simulink model "MRAS_IR2_Ld_Lq_U_comp_dt2_new"  (R2018a)
settings: Solver=ode23t  StartTime=0.0  StopTime=0.3  MaxStep=1e-5  RelTol=1e-4  EnableMultiTasking=on
libraries: powerlib x10, powerlib_meascontrol x10, simulink x1
settings Model: Creator=Алексей  LastModifiedBy=Len_comp
settings SolverCC: ZeroCrossControl=DisableAll  ZeroCrossAlgorithm=Adaptive
settings DataIOCC: SaveFormat=Array  SaveOutput=off  DSMLogging=off  SaveTime=off
settings OptimizationCC: LifeSpan=inf
settings DebuggingCC: UnderspecifiedInitializationDetection=Classic  MergeDetectMultiDrivingBlocksExec=none  SolverPrmCheckMsg=warning  AllowSymbolicDim=off  SFUnexpectedBacktrackingDiag=warning  SFNoUnconditionalDefaultTransitionDiag=warning  SFExecutionAtInitializationDiag=none
settings HardwareCC: ProdBitPerPointer=32  ProdBitPerSizeT=32  ProdBitPerPtrDiffT=32  ProdLargestAtomicFloat=None  ProdIntDivRoundTo=Undefined  ProdEndianess=Unspecified  ProdWordSize=32  ProdHWDeviceType=32-bit Generic
settings ModelReferenceCC: PropagateSignalLabelsOutOfModel=off
settings CodeAppCC: StateflowObjectComments=on
settings GRTTargetCC: TargetLangStandard=C89/C90 (ANSI)  GeneratePreprocessorConditionals=Disable all
settings ConfigComp: CovMetricSettings=dw  CovHtmlReporting=on  CovSaveCumulativeToWorkspaceVar=on  CovSaveSingleToWorkspaceVar=on  CovExternalEMLEnable=off  CovSFcnEnable=off
settings SimscapeCC: SimscapeNormalizeSystem=off

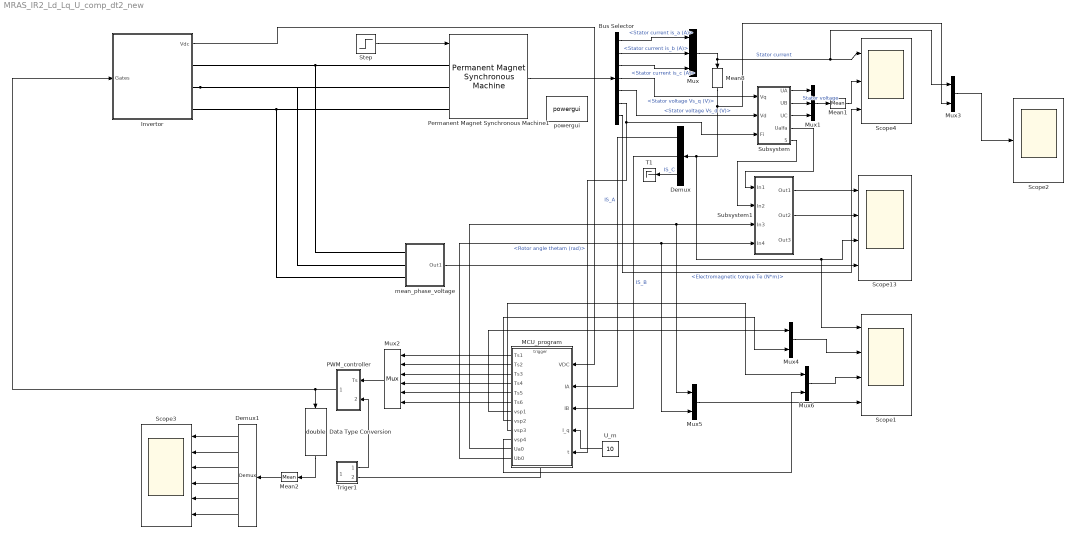
== system MRAS_IR2_Ld_Lq_U_comp_dt2_new ==
  Bus Selector : BusSelector  OutputSignals=Stator current is_a (A),Stator current is_b (A),Stator current is_c (A),Stator voltage Vs_q (V),Stator voltage Vs_d (V),Rotor angle thetam (rad),Electromagnetic torque Te (N*m)
  Data Type Conversion : DataTypeConversion  OutDataTypeStr=double
  Demux : Demux  Outputs=3
  Demux1 : Demux  Outputs=6
  Invertor : Subsystem
  MCU_program : MATLAB Function  TreatAsAtomicUnit=on
  Mean1 : powerlib_meascontrol/Measurements/Mean  Freq=10000  Vinit=0  Ts=0
  Mean2 : powerlib_meascontrol/Measurements/Mean  Freq=10000  Vinit=0  Ts=0
  Mean8 : powerlib_meascontrol/Measurements/Mean  Freq=20000  Vinit=0  Ts=0
  Mux : Mux  Inputs=3
  Mux1 : Mux  Inputs=3
  Mux2 : Mux  Inputs=6
  Mux{3..6} (4 alike) : Mux  Inputs=2
  PWM_controller : Subsystem
  Permanent Magnet Synchronous Machine1 : powerlib/Machines/Permanent Magnet Synchronous Machine  NbPhases=3  FluxDistribution=Sinusoidal  RotorType=Round  MechanicalLoad=Speed w  PresetModel=No  ShowDetailedParameters=on  MeasurementBus=off  Resistance=0.04  Inductance=8.5e-3  dqInductances=[44e-3,39.8e-3]  La=15e-6  MachineConstant=Flux linkage established by magnets (V.s)  Flux=0.0345  VoltageCst=6.2576  TorqueCst=0.05175  Flat=120  Mechanical=[2e4 3e-03 1 0]  PolePairs=1  InitialConditions=[0,0, 0,0]  InitialConditions5ph=[0 0 0 0 0 0]  TsPowergui=0  TsBlock=-1  RefAngle=Aligned with phase A axis (original Park)
      settings: SourceProductName=Simscape Power Systems
  Scope1 : Scope  NumInputPorts=4
  Scope13 : Scope  NumInputPorts=4
  Scope2 : Scope
  Scope3 : Scope  NumInputPorts=6
  Scope4 : Scope  NumInputPorts=3
  Step : Step  Time=0.025  Before=500  After=50  SampleTime=0
  Subsystem : Subsystem
  Subsystem1 : Subsystem
  T1 : Terminator
  Triger1 : Subsystem
  U_m : Constant  Value=10
  mean_phase_voltage : Subsystem
  powergui : powerlib/powergui  Priority=1  SimulationMode=Continuous  SampleTime=50e-6  frequency=60  Iterations=50  frequencyindice=0  Pbase=100e6  ErrMax=1e-4  UnitsV=kV  UnitsW=MW  buscounter=0  FunctionMessages=off  echomessages=off  EnableUseOfTLC=off  CurrentSourceSwitches=on  DisableSnubberDevices=off  DisableRonSwitches=off  DisableVfSwitches=off  DisplayEquations=off  SolverType=Tustin  Interpol=off  ExternalGateDelay=off  methode=off  Ts=0  x0status=blocks  SPID=off  SwTol=0  HookPort=off  RestoreLinks=warning  ResistiveCurrentMeasurement=off  Frange=[0:2:500]  Ylog=off  Xlog=on  ShowGrid=off  save=off  variable=ZData  structure=SD2  ZoomFFT=on  StartTime=0.7  cycles=10  DisplayStyle=4  fundamental=382  FreqAxis=off  MaxFrequency=50000  frequencyindicesteady=1  RmsSteady=1  display=off
  wires:
  Demux/1 -> MCU_program/2(IA)  "IS_A"
  Demux/2 -> MCU_program/3(IB)  "IS_B"
  Permanent Magnet Synchronous Machine1/1 -> Bus Selector/1
  Bus Selector/1 -> Mux/1  "<Stator current is_a (A)>"
  Bus Selector/2 -> Mux/2  "<Stator current is_b (A)>"
  Bus Selector/3 -> Mux/3  "<Stator current is_c (A)>"
  Bus Selector/4 -> Subsystem/1(Vq)  "<Stator voltage Vs_q (V)>"
  Bus Selector/5 -> Subsystem/2(Vd)  "<Stator voltage Vs_d (V)>"
  Subsystem/2(UB) -> Mux1/2
  Subsystem/3(UC) -> Mux1/3
  Subsystem/1(UA) -> Mux1/1
  Mux/1 -> Mean8/1, Mux3/1, Scope4/1  "Stator current"
  Mux1/1 -> Mean1/1  "Stator voltage"
  Step/1 -> Permanent Magnet Synchronous Machine1/1
  MCU_program/1(Ts1) -> Mux2/1
  MCU_program/2(Ts2) -> Mux2/2
  MCU_program/3(Ts3) -> Mux2/3
  MCU_program/4(Ts4) -> Mux2/4
  MCU_program/5(Ts5) -> Mux2/5
  MCU_program/6(Ts6) -> Mux2/6
  Mux2/1 -> PWM_controller/1(Ts)
  Triger1/1(1) -> PWM_controller/2(pila)
  PWM_controller/1(Tss) -> Invertor/1(Gates), Data Type Conversion/1
  Triger1/2(2) -> MCU_program/Trigger
  Invertor/1(Vdc) -> MCU_program/1(VDC)
  Demux/3 -> T1/1  "IS_C"
  U_m/1 -> MCU_program/4(I_q)
  Mean8/1 -> Mux3/2, Scope1/1, Scope13/3, Demux/1
  Demux1/1 -> Scope3/1
  Demux1/3 -> Scope3/3
  Demux1/2 -> Scope3/2
  Demux1/4 -> Scope3/4
  Demux1/5 -> Scope3/5
  Demux1/6 -> Scope3/6
  mean_phase_voltage/1(Out1) -> Scope13/4
  Subsystem/4(Ualfa) -> Subsystem1/1(In1)
  Subsystem/5(Ubeta) -> Subsystem1/2(In2)
  MCU_program/11(Ua0) -> Mux5/1, Subsystem1/3(In3)
  MCU_program/12(Ub0) -> Subsystem1/4(In4), Mux5/2
  Subsystem1/1(Out1) -> Scope13/1
  Subsystem1/2(Out2) -> Scope13/2
  MCU_program/7(vsp1) -> Mux4/1
  MCU_program/8(vsp2) -> Mux4/2
  MCU_program/9(vsp3) -> Mux6/1
  Mux3/1 -> Scope2/1
  Mean1/1 -> Scope4/2
  Mean2/1 -> Demux1/1
  Data Type Conversion/1 -> Mean2/1
  MCU_program/10(vsp4) -> Mux6/2
  Mux5/1 -> Scope1/4
  Mux6/1 -> Scope1/3
  Mux4/1 -> Scope1/2
  Bus Selector/6 -> Subsystem/3(Fi), MCU_program/5(t)  "<Rotor angle thetam (rad)>"
  Bus Selector/7 -> Scope4/3  "<Electromagnetic torque Te (N*m)>"
  connections:
  Permanent Magnet Synchronous Machine1/LConn1 -- mean_phase_voltage/LConn1 -- Invertor/RConn1
  Invertor/RConn2 -- mean_phase_voltage/LConn2 -- Permanent Magnet Synchronous Machine1/LConn2
  Invertor/RConn3 -- mean_phase_voltage/LConn3 -- Permanent Magnet Synchronous Machine1/LConn3

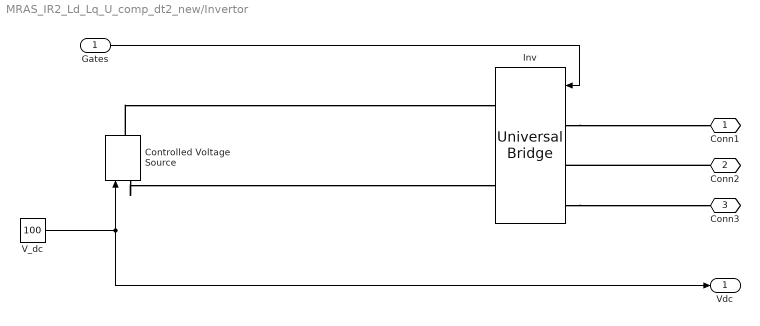
== system MRAS_IR2_Ld_Lq_U_comp_dt2_new/Invertor ==
  Gates : Inport
  Controlled Voltage Source : powerlib/Electrical Sources/Controlled Voltage Source  Initialize=on  Source_Type=AC  Amplitude=0  Phase=0  Frequency=0  Measurements=None
  Inv : powerlib/Power Electronics/Universal Bridge  Arms=3  SnubberResistance=1e9  SnubberCapacitance=inf  Device=IGBT / Diodes  Ron=1e-6  Lon=0  ForwardVoltages="[  0 0  ]"  ForwardVoltage=0  GTOparameters=[ 10e-6 , 20e-6 ]  IGBTparameters=[ 1e-7 , 1e-7 ]  Measurements=None  Measurements_2=None  converterType=Rectifier
  "V_dc " : Constant  Value=100
  Conn1 : PMIOPort  Side=Right
  Conn2 : PMIOPort  Port=2  Side=Right
  Conn3 : PMIOPort  Port=3  Side=Right
  Vdc : Outport
  wires:
  Gates/1 -> Inv/1
  "V_dc "/1 -> Controlled Voltage Source/1, Vdc/1
  connections:
  Controlled Voltage Source/RConn1 -- Inv/RConn1
  Conn2/RConn1 -- Inv/LConn2
  Controlled Voltage Source/LConn1 -- Inv/RConn2
  Inv/LConn3 -- Conn3/RConn1
  Inv/LConn1 -- Conn1/RConn1

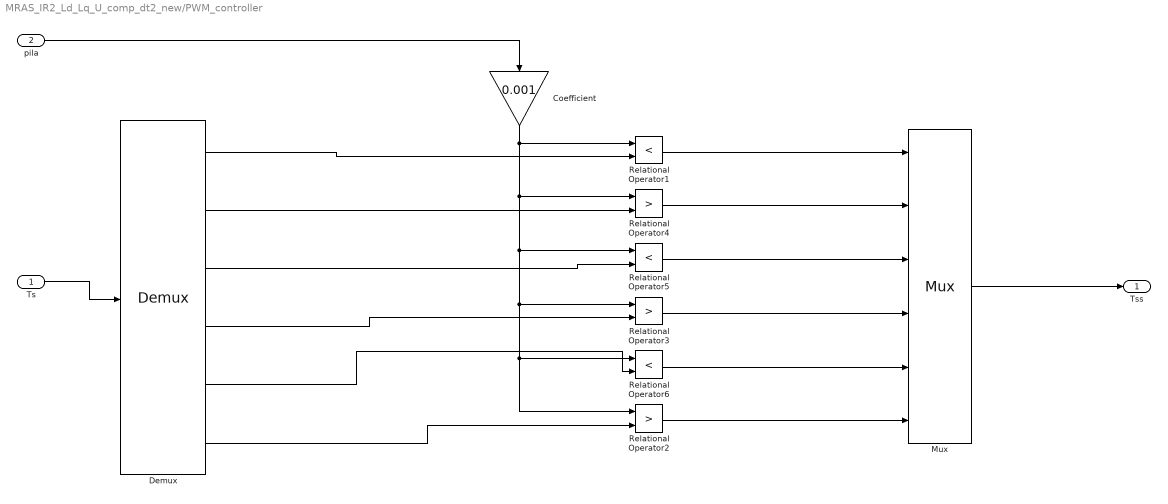
== system MRAS_IR2_Ld_Lq_U_comp_dt2_new/PWM_controller ==
  Ts : Inport
  pila : Inport  Port=2
  Coefficient : Gain  Gain=0.001
  Demux : Demux  Outputs=6
  Mux : Mux  Inputs=6
  Relational Operator1 : RelationalOperator  Operator=<  OutDataTypeStr=boolean  RndMeth=Nearest
  Relational Operator2 : RelationalOperator  Operator=>  OutDataTypeStr=boolean  RndMeth=Nearest
  Relational Operator3 : RelationalOperator  Operator=>  OutDataTypeStr=boolean  RndMeth=Nearest
  Relational Operator4 : RelationalOperator  Operator=>  OutDataTypeStr=boolean  RndMeth=Nearest
  Relational Operator5 : RelationalOperator  Operator=<  OutDataTypeStr=boolean  RndMeth=Nearest
  Relational Operator6 : RelationalOperator  Operator=<  OutDataTypeStr=boolean  RndMeth=Nearest
  Tss : Outport
  wires:
  Relational Operator4/1 -> Mux/2
  Demux/4 -> Relational Operator3/2
  Demux/6 -> Relational Operator2/2
  Relational Operator3/1 -> Mux/4
  Relational Operator2/1 -> Mux/6
  Ts/1 -> Demux/1
  Coefficient/1 -> Relational Operator3/1, Relational Operator2/1, Relational Operator6/1, Relational Operator5/1, Relational Operator4/1, Relational Operator1/1
  Relational Operator1/1 -> Mux/1
  Relational Operator5/1 -> Mux/3
  Relational Operator6/1 -> Mux/5
  Demux/1 -> Relational Operator1/2
  Demux/3 -> Relational Operator5/2
  Demux/5 -> Relational Operator6/2
  Demux/2 -> Relational Operator4/2
  pila/1 -> Coefficient/1
  Mux/1 -> Tss/1

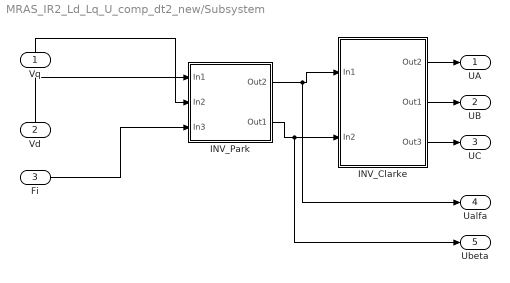
== system MRAS_IR2_Ld_Lq_U_comp_dt2_new/Subsystem ==
  Vq : Inport
  Vd : Inport  Port=2
  Fi : Inport  Port=3
  INV_Clarke : Subsystem
  INV_Park : Subsystem
  UA : Outport
  UB : Outport  Port=2
  UC : Outport  Port=3
  Ualfa : Outport  Port=4
  Ubeta : Outport  Port=5
  wires:
  INV_Clarke/2(Out1) -> UB/1
  INV_Park/1(Out2) -> Ualfa/1, INV_Clarke/1(In1)
  INV_Clarke/1(Out2) -> UA/1
  INV_Park/2(Out1) -> Ubeta/1, INV_Clarke/2(In2)
  INV_Clarke/3(Out3) -> UC/1
  Fi/1 -> INV_Park/3(In3)
  Vd/1 -> INV_Park/1(In1)
  Vq/1 -> INV_Park/2(In2)

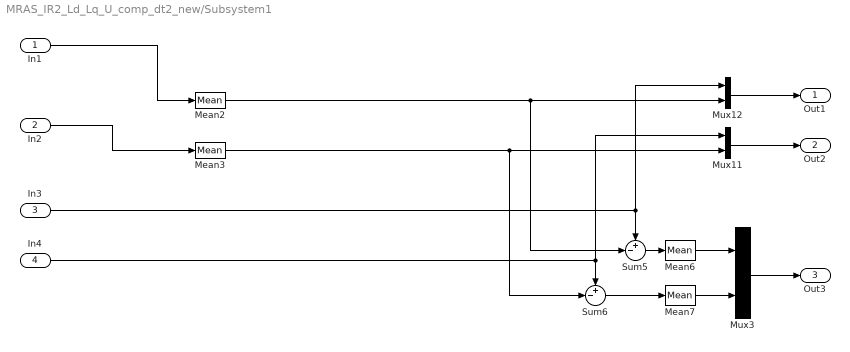
== system MRAS_IR2_Ld_Lq_U_comp_dt2_new/Subsystem1 ==
  In1 : Inport
  In2 : Inport  Port=2
  In3 : Inport  Port=3
  In4 : Inport  Port=4
  Mean2 : powerlib_meascontrol/Measurements/Mean  Freq=10000  Vinit=0  Ts=0
  Mean3 : powerlib_meascontrol/Measurements/Mean  Freq=10000  Vinit=0  Ts=0
  Mean6 : powerlib_meascontrol/Measurements/Mean  Freq=20000  Vinit=0  Ts=0
  Mean7 : powerlib_meascontrol/Measurements/Mean  Freq=20000  Vinit=0  Ts=0
  Mux11 : Mux  Inputs=2
  Mux12 : Mux  Inputs=2
  Mux3 : Mux  Inputs=2
  Sum5 : Sum  Inputs=+-|
  Sum6 : Sum  Inputs=+-|
  Out1 : Outport
  Out2 : Outport  Port=2
  Out3 : Outport  Port=3
  wires:
  In4/1 -> Mux11/1, Sum6/1
  Mean7/1 -> Mux3/2
  Sum6/1 -> Mean7/1
  Mean2/1 -> Sum5/2, Mux12/2
  Mean3/1 -> Sum6/2, Mux11/2
  Mean6/1 -> Mux3/1
  Mux11/1 -> Out2/1
  Sum5/1 -> Mean6/1
  In3/1 -> Sum5/1, Mux12/1
  In1/1 -> Mean2/1
  In2/1 -> Mean3/1
  Mux12/1 -> Out1/1
  Mux3/1 -> Out3/1

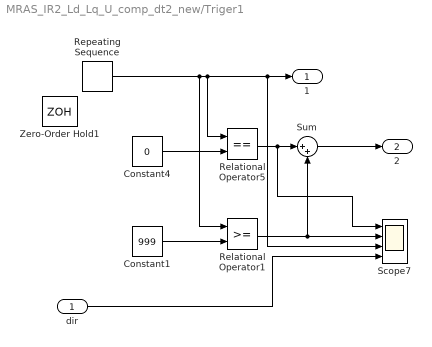
== system MRAS_IR2_Ld_Lq_U_comp_dt2_new/Triger1 ==
  dir : Inport
  Constant1 : Constant  Value=999
  Constant4 : Constant  Value=0
  Relational Operator1 : RelationalOperator  OutDataTypeStr=boolean  RndMeth=Nearest
  Relational Operator5 : RelationalOperator  Operator===  OutDataTypeStr=boolean  RndMeth=Nearest
  Repeating Sequence : simulink/Sources/Repeating Sequence  rep_seq_t=[0 2.5e-5 5e-5]  rep_seq_y=[0 1000 0]
  Scope7 : Scope  NumInputPorts=4
  Sum : Sum  Inputs=|++
  Zero-Order Hold1 : ZeroOrderHold  SampleTime=5e-9
  1 : Outport
  2 : Outport  Port=2
  wires:
  Repeating Sequence/1 -> Relational Operator1/1, Relational Operator5/1, Scope7/3, 1/1
  Constant4/1 -> Relational Operator5/2
  Sum/1 -> 2/1
  Constant1/1 -> Relational Operator1/2
  Relational Operator5/1 -> Scope7/1, Sum/1
  Relational Operator1/1 -> Scope7/2, Sum/2
  dir/1 -> Scope7/4

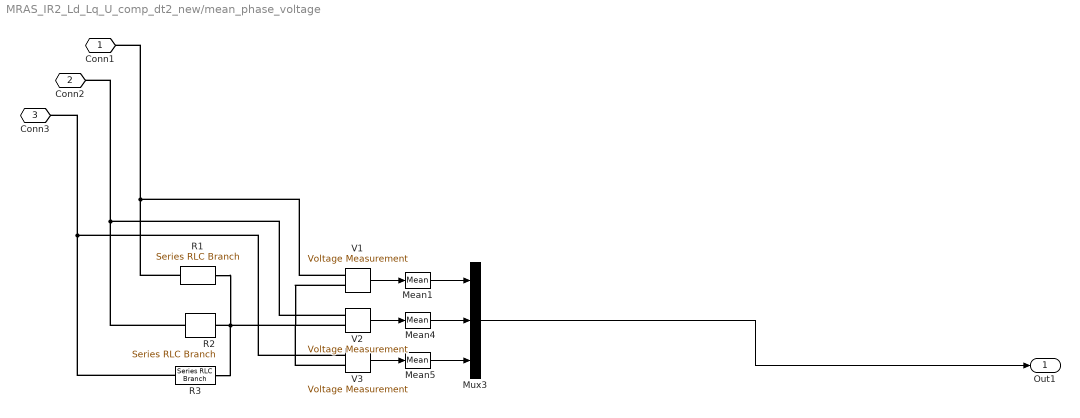
== system MRAS_IR2_Ld_Lq_U_comp_dt2_new/mean_phase_voltage ==
  Mean1 : powerlib_meascontrol/Measurements/Mean  Freq=10000  Vinit=0  Ts=0
  Mean4 : powerlib_meascontrol/Measurements/Mean  Freq=10000  Vinit=0  Ts=0
  Mean5 : powerlib_meascontrol/Measurements/Mean  Freq=10000  Vinit=0  Ts=0
  Mux3 : Mux  Inputs=3
  R1 : powerlib/Elements/Series RLC Branch  LConnTagsString=__new0  RConnTagsString=__new0  BranchType=R  Resistance=1e6  Inductance=1e-3  SetiL0=off  InitialCurrent=0  Capacitance=1e-6  Setx0=off  InitialVoltage=0  Measurements=None
  R2 : powerlib/Elements/Series RLC Branch  LConnTagsString=__new0  RConnTagsString=__new0  BranchType=R  Resistance=1e6  Inductance=1e-3  SetiL0=off  InitialCurrent=0  Capacitance=1e-6  Setx0=off  InitialVoltage=0  Measurements=None
  R3 : powerlib/Elements/Series RLC Branch  LConnTagsString=__new0  RConnTagsString=__new0  BranchType=R  Resistance=1e6  Inductance=1e-3  SetiL0=off  InitialCurrent=0  Capacitance=1e-6  Setx0=off  InitialVoltage=0  Measurements=None
  V1 : powerlib/Measurements/Voltage Measurement  PhasorSimulation=off  OutputType=Complex  PSBequivalent=0
  V2 : powerlib/Measurements/Voltage Measurement  PhasorSimulation=off  OutputType=Complex  PSBequivalent=0
  V3 : powerlib/Measurements/Voltage Measurement  PhasorSimulation=off  OutputType=Complex  PSBequivalent=0
  Conn1 : PMIOPort  Side=Left
  Conn2 : PMIOPort  Port=2  Side=Left
  Conn3 : PMIOPort  Port=3  Side=Left
  Out1 : Outport
  wires:
  V2/1 -> Mean4/1
  Mean1/1 -> Mux3/1
  V3/1 -> Mean5/1
  Mean4/1 -> Mux3/2
  Mean5/1 -> Mux3/3
  V1/1 -> Mean1/1
  Mux3/1 -> Out1/1
  connections:
  R3/LConn1 -- Conn3/RConn1 -- V3/LConn1
  R2/LConn1 -- Conn2/RConn1 -- V2/LConn1
  R3/RConn1 -- V3/LConn2 -- V1/LConn2 -- V2/LConn2 -- R1/RConn1 -- R2/RConn1
  R1/LConn1 -- Conn1/RConn1 -- V1/LConn1

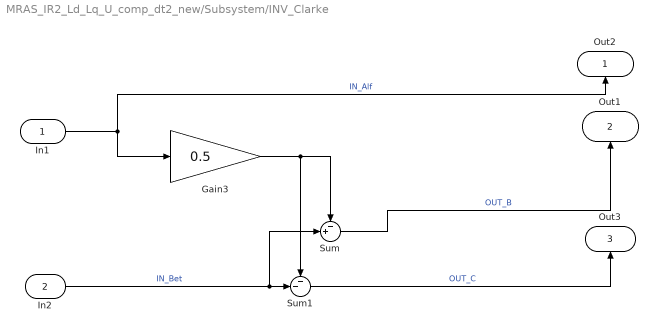
== system MRAS_IR2_Ld_Lq_U_comp_dt2_new/Subsystem/INV_Clarke ==
  In1 : Inport
  In2 : Inport  Port=2
  Gain3 : Gain  Gain=0.5
  Sum : Sum  Inputs=-+|
  Sum1 : Sum  Inputs=--|
  Out2 : Outport
  Out1 : Outport  Port=2
  Out3 : Outport  Port=3
  wires:
  Sum/1 -> Out1/1  "OUT_B"
  In2/1 -> Sum/2, Sum1/2  "IN_Bet"
  In1/1 -> Out2/1, Gain3/1  "IN_Alf"
  Sum1/1 -> Out3/1  "OUT_C"
  Gain3/1 -> Sum1/1, Sum/1

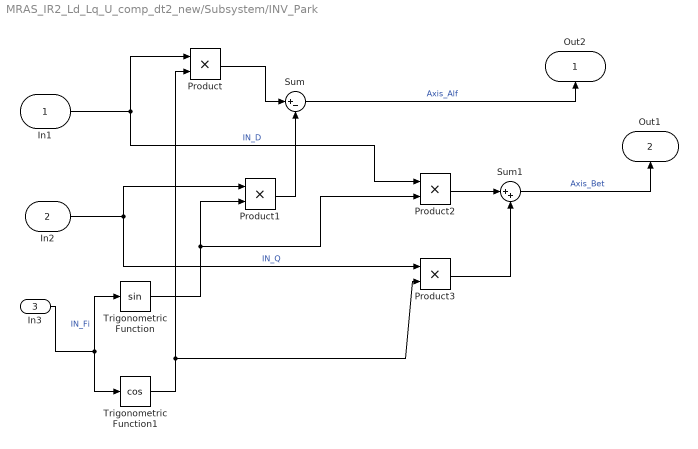
== system MRAS_IR2_Ld_Lq_U_comp_dt2_new/Subsystem/INV_Park ==
  In1 : Inport
  In2 : Inport  Port=2
  In3 : Inport  Port=3
  Product{,1..3} (4 alike) : Product
  Sum : Sum  Inputs=|+-
  Sum1 : Sum  Inputs=|++
  Trigonometric Function : Trigonometry
  Trigonometric Function1 : Trigonometry  Operator=cos
  Out2 : Outport
  Out1 : Outport  Port=2
  wires:
  Sum1/1 -> Out1/1  "Axis_Bet"
  In2/1 -> Product1/1, Product3/1  "IN_Q"
  In1/1 -> Product2/1, Product/1  "IN_D"
  Sum/1 -> Out2/1  "Axis_Alf"
  In3/1 -> Trigonometric Function1/1, Trigonometric Function/1  "IN_Fi"
  Trigonometric Function1/1 -> Product/2, Product3/2
  Trigonometric Function/1 -> Product2/2, Product1/2
  Product1/1 -> Sum/2
  Product/1 -> Sum/1
  Product2/1 -> Sum1/1
  Product3/1 -> Sum1/2

== matlab function MRAS_IR2_Ld_Lq_U_comp_dt2_new/MCU_program ==
  data: VDC input; IA input; IB input; Ts1 output; Ts2 output; Ts3 output; Ts4 output; Ts5 output; Ts6 output; I_q input; vsp1 output; vsp2 output; vsp3 output; vsp4 output; Ua0 output; Ub0 output; t input
  events: trigger input RISING_EDGE_EVENT
function [Ts1,Ts2,Ts3,Ts4,Ts5,Ts6,vsp1,vsp2,vsp3,vsp4,Ua0,Ub0] = fcn(VDC,IA,IB,I_q,t)
%время 1/2 ШИМ периода
dt=25e-6;

dead=0.00;
dtc =0.00;
dtc=dtc/(dt*1e6);

Uvt=0;
Uvd=0;
w=50;

kuqp =0.5;
kudp =0.5;
kuqi =1333;
kudi =1333;

%persistent tet;
persistent dir;
persistent IAp;
persistent IBp;
persistent ICp;

persistent Udint;
persistent Uqint;

%заполнение начальных значений static переменным (persistent здесь)

%if isempty(tet)
%    tet=pi/2;
%end; 

if isempty(dir)
    dir=1;
end; 
if isempty(IAp)
    IAp=0;
end; 
if isempty(IBp)
    IBp=0;
end; 
if isempty(ICp)
    ICp=0;
end; 
if isempty(Udint)
    Udint=0;
end; 
if isempty(Uqint)
    Uqint=0;
end; 




%tet=tet+w*dt;
tet = t;
while (tet > 2*pi)
    tet = tet-2*pi;
end;

Ialfa=IA;
Ibeta=(2*IB+IA)/1.7320508;
Id=Ialfa*cos(tet)+Ibeta*sin(tet);
Iq=Ibeta*cos(tet)-Ialfa*sin(tet); 


%ПИ-регулятор для напряжения по оси Ку
diq=I_q-Iq;
Uqpr=diq*kuqp;
Uqint=Uqint+diq*kuqi*dt;
U_q = Uqpr+Uqint;
%ПИ-регулятор для напряжения по оси Дэ
did=0-Id;
Udpr=did*kudp;
Udint=Udint+did*kudi*dt;
U_d = Udpr+Udint;


%U_d = 0;
%U_q = 2;



Ua0=U_d*cos(tet)-U_q*sin(tet);
Ub0=U_d*sin(tet)+U_q*cos(tet);



%Ua0k=Ua0+(SIA-0.5*SIB-0.5*SIC)*(dead/(2*dt*1e6))*VDC*2/3;
%Ub0k=Ub0+(SIB-SIC)*(dead/(2*dt*1e6))*(sqrt(3)/2)*VDC*2/3;
Ua0k=Ua0;
Ub0k=Ub0;

%{
vref1=sqrt(Ua0^2+Ub0^2);

Ua0k=Ua0k+(sign(IA)-0.5*sign(IB)-0.5*sign(-IA-IB))*0.5*Uvd*(2/3-vref1/VDC);
Ub0k=Ub0k+(sign(IB)-sign(-IA-IB))*0.5*Uvd*(2/3-vref1/VDC)*(sqrt(3)/2);

Ua0k=Ua0k+(sign(IA)-0.5*sign(IB)-0.5*sign(-IA-IB))*Uvt*(1/3+0.41*vref1/VDC);
Ub0k=Ub0k+(sign(IB)-sign(-IA-IB))*Uvt*(1/3+0.41*vref1/VDC)*(sqrt(3)/2);
%}


vrefa=sqrt(Ua0k^2+Ub0k^2);

vphase=acos(Ua0k/vrefa)*sign(Ub0k)+(sign(Ub0k)-1)*(-pi);

if(vrefa>(2/3)*VDC)
  vrefa=(2/3)*VDC;
end
%вывод на осциллографы



vsp1=tet;
vsp2=vphase;
vsp3=U_d;
vsp4=U_q;

%алгоритм формирования векторной ШИМ  мертвым веменем dead [мкс]
dead=dead/(dt*1e6);
a=vphase;
v2=vrefa*1.5;

%v2=v2+2;
if a>=0 && a<pi/3 
    n=1;
elseif  a>=pi/3 && a<2*pi/3 
    n=2;
elseif  a>=2*pi/3 && a<pi 
    n=3;
elseif  a>=pi && a<4*pi/3 
    n=4;
elseif  a>=4*pi/3 && a<5*pi/3 
    n=5;
else n=6;

end

a_cor=a-(n-1)*pi/3;

T1 = (v2/VDC)*sin(pi/3-a_cor)/sin(pi/3);
T2 = (v2/VDC)*sin(a_cor)/sin(pi/3);
T0=1-T1-T2;
Ta1=0; Ta3=0; Ta5=0; 
switch n
    case 1
        
        Ta1=T1+T2+T0/2;
        
        Ta3=T2+T0/2;
       
        Ta5=T0/2;
       
    case 2
        
        Ta1=T1+T0/2;
        
        Ta3=T1+T2+T0/2;
    
        Ta5=T0/2;       
        
    case 3
        
        Ta1=T0/2;
       
        Ta3=T1+T2+T0/2;
       
        Ta5=T2+T0/2;    
        
    case 4
        
        Ta1=T0/2;
       
        Ta3=T1+T0/2;
       
        Ta5=T1+T2+T0/2;   
       
    case 5
        
        Ta1=T2+T0/2;
        
        Ta3=T0/2;
        
        Ta5=T1+T2+T0/2;     
        
    case 6
        
        Ta1=T1+T2+T0/2;
        
        Ta3=T0/2;
     
        Ta5=T1+T0/2;    
        
end;

if(IA>-0.0)
    Ta1=(Ta1*VDC+Uvd)/(VDC-Uvt+Uvd);
elseif(IA<=0.0)
    Ta1=(Ta1*VDC-Uvt)/(VDC-Uvt+Uvd);
end;

if(IB>-0.0)
    Ta3=(Ta3*VDC+Uvd)/(VDC-Uvt+Uvd);
elseif(IB<0.0)
    Ta3=(Ta3*VDC-Uvt)/(VDC-Uvt+Uvd);
end;

if((-IA-IB)>-0.0)
    Ta5=(Ta5*VDC+Uvd)/(VDC-Uvt+Uvd);
elseif((-IA-IB)<0.0)
    Ta5=(Ta5*VDC-Uvt)/(VDC-Uvt+Uvd);
end;


Ts1=(Ta1)+dead/2; 
Ts3=(Ta3)+dead/2; 
Ts5=(Ta5)+dead/2;
Ts2=(Ta1)-dead/2; 
Ts4=(Ta3)-dead/2; 
Ts6=(Ta5)-dead/2;

%{
if(dir==1)
    Ts1=(Ta1); 
    Ts3=(Ta3); 
    Ts5=(Ta5);
    Ts2=(Ta1)+dead; 
    Ts4=(Ta3)+dead; 
    Ts6=(Ta5)+dead;
else
    Ts1=(Ta1)-dead; 
    Ts3=(Ta3)-dead; 
    Ts5=(Ta5)-dead;
    Ts2=(Ta1); 
    Ts4=(Ta3); 
    Ts6=(Ta5);    
end;
%}

if (IA>-0.0)
    Ts1=Ts1+dtc/2;
    Ts2=Ts2+dtc/2;
elseif (IA<0.0)
    Ts1=Ts1-dtc/2;
    Ts2=Ts2-dtc/2;           
end;
if (IB>-0.0)
    Ts3=Ts3+dtc/2;
    Ts4=Ts4+dtc/2;
elseif(IB<0.0)
    Ts3=Ts3-dtc/2;
    Ts4=Ts4-dtc/2; 
end;  
if ((-IA-IB)>-0.0)
    Ts5=Ts5+dtc/2;
    Ts6=Ts6+dtc/2;
elseif((-IA-IB)<0.0)
    Ts5=Ts5-dtc/2;
    Ts6=Ts6-dtc/2;           
end;


return;
